simulink model "controller_attitude_pitch"  (R2019b)
settings: Solver=FixedStepAuto  StartTime=0.0  StopTime=10.0  FixedStep=1/sim_freq  RelTol=1e-3
undefined symbols (not defined in the file): G_P_OL_DENOM, G_P_OL_NUM, K_theta, sim_freq
settings Model: Creator=francois  LastModifiedBy=francois

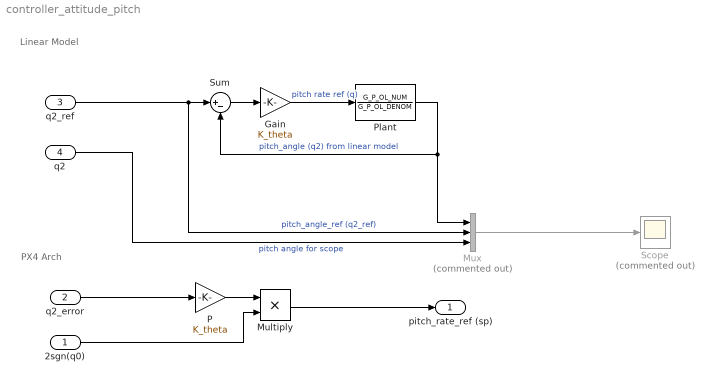
== system controller_attitude_pitch ==
  note: Linear Model
  note: PX4 Arch
  2sgn(q0) : Inport  SampleTime=1/sim_freq
  q2_error : Inport  Port=2  SampleTime=1/sim_freq
  q2_ref : Inport  Port=3
  q2 : Inport  Port=4  SampleTime=1/sim_freq
  Gain : Gain  Gain=K_theta
  Multiply : Product
  Mux : Mux  Commented=on  Inputs=3
  P : Gain  Gain=K_theta
  Plant : TransferFcn  Numerator=G_P_OL_NUM  Denominator=G_P_OL_DENOM
  Scope : Scope  Commented=on
  Sum : Sum  Inputs=|+-
  pitch_rate_ref (sp) : Outport  VectorParamsAs1DForOutWhenUnconnected=off
  wires:
  q2_ref/1 -> Mux/2, Sum/1  "pitch_angle_ref (q2_ref)"
  Plant/1 -> Mux/1, Sum/2  "pitch_angle (q2) from linear model"
  Sum/1 -> Gain/1
  Gain/1 -> Plant/1  "pitch rate ref (q)"
  P/1 -> Multiply/1
  2sgn(q0)/1 -> Multiply/2
  q2_error/1 -> P/1
  Multiply/1 -> pitch_rate_ref (sp)/1
  q2/1 -> Mux/3  "pitch angle for scope"
  Mux/1 -> Scope/1
